simulink model "R_soft_sim"  (R2021a)
settings: Solver=VariableStepAuto  StartTime=0.0  StopTime=10.0  RelTol=1e-3
values from neighbouring files (symbols this model uses):
  m = size(Delta, 2)    [filtration.m]    (also in rowFiltration.m)
undefined symbols (not defined in the file or in its folder): beta, D, g, k, L, theta_dot_init, theta_init
settings Model: Creator=Utente  LastModifiedBy=Utente

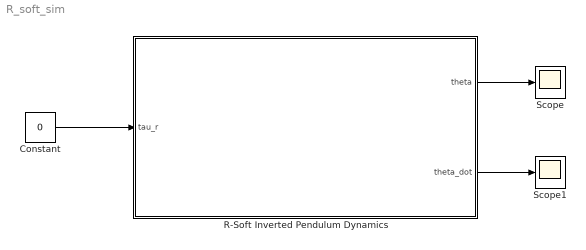
== system R_soft_sim ==
  Constant : Constant  Value=0
  R-Soft Inverted Pendulum Dynamics : Subsystem
  Scope : Scope
  Scope1 : Scope
  wires:
  Constant/1 -> R-Soft Inverted Pendulum Dynamics/1(tau_r)
  R-Soft Inverted Pendulum Dynamics/1(theta) -> Scope/1
  R-Soft Inverted Pendulum Dynamics/2(theta_dot) -> Scope1/1

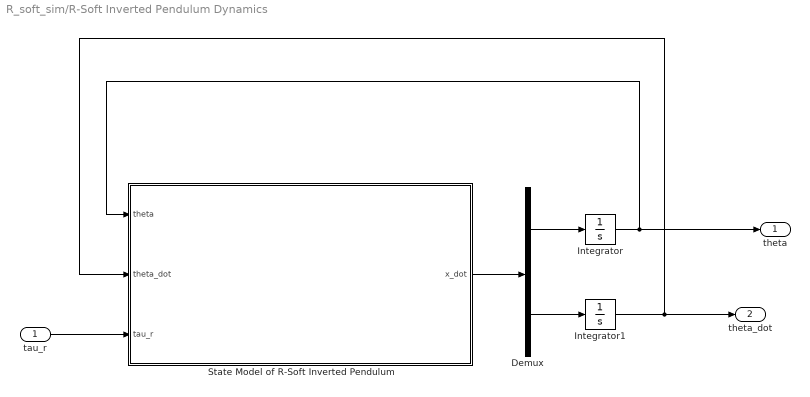
== system R_soft_sim/R-Soft Inverted Pendulum Dynamics ==
  tau_r : Inport
  Demux : Demux  Outputs=2
  Integrator : Integrator  InitialCondition=theta_init
  Integrator1 : Integrator  InitialCondition=theta_dot_init
  State Model of R-Soft Inverted Pendulum : MATLAB Function  TreatAsAtomicUnit=on
  theta : Outport
  theta_dot : Outport  Port=2
  wires:
  tau_r/1 -> State Model of R-Soft Inverted Pendulum/3(tau_r)
  State Model of R-Soft Inverted Pendulum/1(x_dot) -> Demux/1
  Demux/1 -> Integrator/1
  Integrator/1 -> State Model of R-Soft Inverted Pendulum/1(theta), theta/1
  Demux/2 -> Integrator1/1
  Integrator1/1 -> theta_dot/1, State Model of R-Soft Inverted Pendulum/2(theta_dot)

== matlab function R_soft_sim/R-Soft Inverted Pendulum Dynamics/State Model of R-Soft Inverted Pendulum ==
  data: theta input; x_dot output; theta_dot input; tau_r input; m parameter; L parameter; D parameter; g parameter; k parameter; beta parameter
function x_dot = state_model(theta, theta_dot, tau_r, m, L, D, g, k, beta)
x1 = theta;
x2 = theta_dot;

B = inertiaMatrix(theta(1), theta(2), theta(3), m, L, D);
G = gravityVector(theta(1), theta(2), theta(3), m, g, L, D);
C = coriolisMatrix(theta(1), theta(2), theta(3), theta_dot(1), theta_dot(2), theta_dot(3), m, L, D);
K = elasticMatrix(k);
D = dampingMatrix(beta);

f = [x2; -inv(B)*(C*x2 + G + K*x1 + D*x2)];
g = [zeros(3, 1); inv(B)*[1; 0; 0]];

x_dot = f + g*tau_r;
end
